simulink model "teste_simulink"  (R2015b)
settings: Solver=VariableStepAuto  StartTime=0.0  StopTime=10  FixedStep=0.002  RelTol=1e-3
settings Model: ExtModeTrigDuration=5000  Creator=UFRN  LastModifiedBy=UFRN
settings SolverCC: PositivePriorityOrder=on
settings RTWCC: SystemTargetFile=quarc_win64.tlc  TemplateMakefile=quarc_default_tmf  Description=QUARC Win64 Target
settings STFCustomTargetCC: GeneratePreprocessorConditionals=Use local settings  CPPClassGenCompliant=off
settings GRTTargetCC: ParMdlRefBuildCompliant=off  CompOptLevelCompliant=off  CombineOutputUpdateFcns=off  MatFileLogging=off  CPPClassGenCompliant=off  GRTInterface=on  UseToolchainInfoCompliant=off  ExtMode=on  ExtModeMexFile=quarc_comm

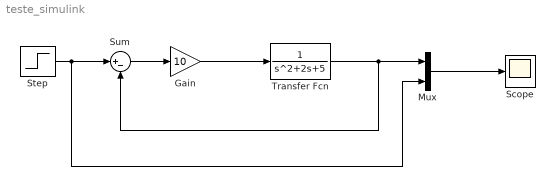
== system teste_simulink ==
  Gain : Gain  Gain=10
  Mux : Mux  Inputs=2
  Scope : Scope
  Step : Step  Time=0  SampleTime=0
  Sum : Sum  Inputs=|+-
  Transfer Fcn : TransferFcn  Denominator=[1 2 5]
  wires:
  Mux/1 -> Scope/1
  Transfer Fcn/1 -> Sum/2, Mux/1
  Gain/1 -> Transfer Fcn/1
  Sum/1 -> Gain/1
  Step/1 -> Sum/1, Mux/2
